simulink model "AMT103"  (R2024b)
settings: Solver=FixedStepAuto  StartTime=0.0  StopTime=inf  FixedStep=0.001  RelTol=1e-3  EnableMultiTasking=on
libraries: stm32f4xxblockslib x3, stm32g4xxblockslib x3, simulink x1
settings Model: STM32="{\"DigitalPortRead\":[{\"ID\":\"e:8\"},{\"ID\":\"e:9\"},{\"ID\":\"e:38\"},{\"ID\":\"e:39\"},{\"ID\":\"AMT103:38\"},{\"ID\":\"AMT103:9\"},{\"ID\":\"AMT103:8\"}],\"EncoderBlockForG4\":[{\"ID\":\"e:26\"},{\"ID\":\"e:27\"},{\"ID\":\"e:28\"},{\"ID\":\"AMT103:26\"},{\"ID\":\"AMT103:27\"},{\"ID\":\"AMT103:28\"}]}"  SimulationMode=external  Creator=gamen  LastModifiedBy=gamen
settings OptimizationCC: DefaultParameterBehavior=Inlined  EnhancedBackFolding=on  PassReuseOutputArgsAs=Individual arguments  ZeroExternalMemoryAtStartup=off  ZeroInternalMemoryAtStartup=off  MaxStackSize=512  OptimizeBlockOrder=speed  DifferentSizesBufferReuse=on  OptimizationCustomize=off  EfficientTunableParamExpr=on
settings DebuggingCC: ParameterTunabilityLossMsg=error
settings HardwareCC: ProdBitPerPointer=32  ProdBitPerSizeT=32  ProdBitPerPtrDiffT=32  ProdLargestAtomicInteger=Long  ProdLargestAtomicFloat=Double  ProdWordSize=32  ProdLongLongMode=on  ProdHWDeviceType=ARM Compatible->ARM Cortex-M
settings SFSimCC: MATLABDynamicMemAlloc=off
settings RTWCC: Description=Embedded Coder  SystemTargetFile=ert.tlc  HardwareBoard=STM32G4xx Based  TemplateMakefile=ert_default_tmf  Toolchain=GNU Tools for ARM Embedded Processors
settings CodeAppCC: ForceParamTrailComments=on  IgnoreCustomStorageClasses=off  OperatorAnnotations=on  SimulinkDataObjDesc=on  SFDataObjDesc=on  InsertBlockDesc=on
settings ERTTargetCC: TargetLangStandard=C99 (ISO)  CodeReplacementLibrary=ARM Cortex-M  ExtModeTransport=3  ExtModeStaticAlloc=on  ExtModeStaticAllocSize=2048  ExtModeMexFile=ext_xcp  ExtModeIntrfLevel=Level2 - Open

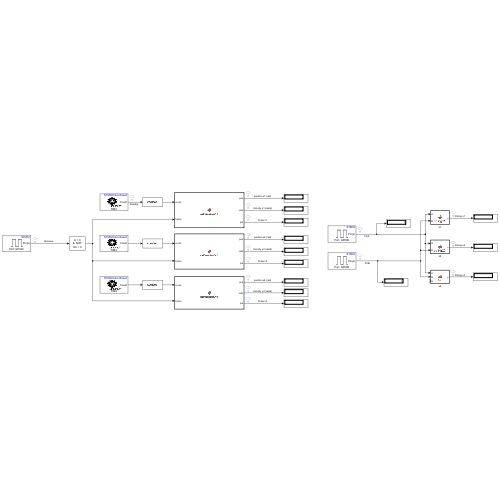
[thumbnail: Simulink's stored preview of the top-level diagram]
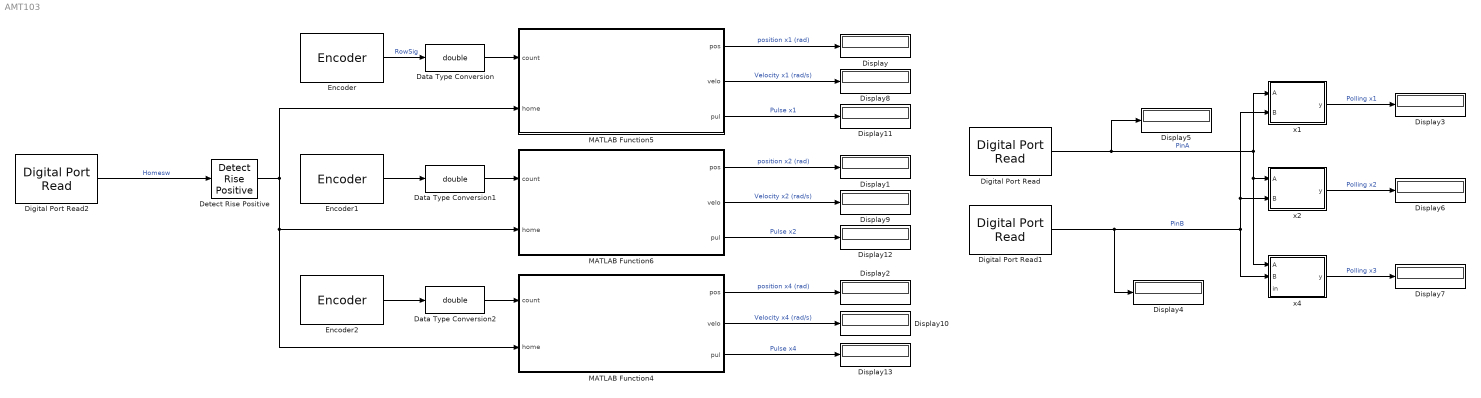
== system AMT103 ==
  Data Type Conversion : DataTypeConversion  OutDataTypeStr=double  SaturateOnIntegerOverflow=off  RndMeth=Floor
  Data Type Conversion1 : DataTypeConversion  OutDataTypeStr=double  SaturateOnIntegerOverflow=off  RndMeth=Floor
  Data Type Conversion2 : DataTypeConversion  OutDataTypeStr=double  SaturateOnIntegerOverflow=off  RndMeth=Floor
  Detect Rise Positive : simulink/Logic and Bit Operations/Detect Rise Positive  vinit=0  OutDataTypeStr=boolean
  Digital Port Read : stm32f4xxblockslib/Digital Port Read  PortName=GPIOB  PinNumber=[4]  ReadOperation=on  IOAsArray=on  SampleTime=-1  EnableSimPort=off  hoistedMaskSrc=ECSoC/ECSimCodegen/Digital Port Read
      settings: LibrarySourceBlock=stm32g4xxblockslib/Digital Port Read
  Digital Port Read1 : stm32f4xxblockslib/Digital Port Read  PortName=GPIOB  PinNumber=[5]  ReadOperation=on  IOAsArray=on  SampleTime=-1  EnableSimPort=off  hoistedMaskSrc=ECSoC/ECSimCodegen/Digital Port Read
      settings: LibrarySourceBlock=stm32g4xxblockslib/Digital Port Read
  Digital Port Read2 : stm32f4xxblockslib/Digital Port Read  PortName=GPIOC  PinNumber=[13]  ReadOperation=on  IOAsArray=on  SampleTime=-1  EnableSimPort=off  hoistedMaskSrc=ECSoC/ECSimCodegen/Digital Port Read
      settings: LibrarySourceBlock=stm32g4xxblockslib/Digital Port Read
  Display{,1..13} (14 alike) : Display
  Encoder : stm32g4xxblockslib/Encoder  TimerModule=TIM3  EnableResetInput=off  OutputCountAfterFirstIndex=off  OutputValidIndex=off  OutputDirection=off  OutputStatus=off  SampleTime=-1
  Encoder1 : stm32g4xxblockslib/Encoder  TimerModule=TIM4  EnableResetInput=off  OutputCountAfterFirstIndex=off  OutputValidIndex=off  OutputDirection=off  OutputStatus=off  SampleTime=-1
  Encoder2 : stm32g4xxblockslib/Encoder  TimerModule=TIM8  EnableResetInput=off  OutputCountAfterFirstIndex=off  OutputValidIndex=off  OutputDirection=off  OutputStatus=off  SampleTime=-1
  MATLAB Function4 : MATLAB Function  TreatAsAtomicUnit=on
  MATLAB Function5 : MATLAB Function  TreatAsAtomicUnit=on
  MATLAB Function6 : MATLAB Function  TreatAsAtomicUnit=on
  x1 : MATLAB Function  TreatAsAtomicUnit=on
  x2 : MATLAB Function  TreatAsAtomicUnit=on
  x4 : MATLAB Function  TreatAsAtomicUnit=on
  wires:
  MATLAB Function6/1(pos) -> Display1/1  "position x2 (rad)"
  Encoder2/1 -> Data Type Conversion2/1
  x2/1(y) -> Display6/1  "Polling x2"
  x4/1(y) -> Display7/1  "Polling x3"
  MATLAB Function5/1(pos) -> Display/1  "position x1 (rad)"
  MATLAB Function6/2(velo) -> Display9/1  "Velocity x2 (rad/s)"
  Data Type Conversion/1 -> MATLAB Function5/1(count)
  MATLAB Function4/3(pul) -> Display13/1  "Pulse x4"
  Encoder/1 -> Data Type Conversion/1  "RowSig"
  Data Type Conversion2/1 -> MATLAB Function4/1(count)
  Digital Port Read1/1 -> x1/2(B), x2/2(B), x4/2(B), Display4/1  "PinB"
  Data Type Conversion1/1 -> MATLAB Function6/1(count)
  MATLAB Function4/1(pos) -> Display2/1  "position x4 (rad)"
  MATLAB Function6/3(pul) -> Display12/1  "Pulse x2"
  Digital Port Read/1 -> Display5/1, x1/1(A), x4/1(A), x2/1(A)  "PinA"
  x1/1(y) -> Display3/1  "Polling x1"
  MATLAB Function5/2(velo) -> Display8/1  "Velocity x1 (rad/s)"
  MATLAB Function4/2(velo) -> Display10/1  "Velocity x4 (rad/s)"
  MATLAB Function5/3(pul) -> Display11/1  "Pulse x1"
  Encoder1/1 -> Data Type Conversion1/1
  Digital Port Read2/1 -> Detect Rise Positive/1  "Homesw"
  Detect Rise Positive/1 -> MATLAB Function5/2(home), MATLAB Function4/2(home), MATLAB Function6/2(home)

== matlab function AMT103/x1 ==
  data: A input; y output; B input
function y =  pollingX1(A, B)
    persistent c stageA
    if isempty(c)
        c = 0;
        stageA = 1;
    end

    if A == 0 && stageA
        stageA = 0;
        c = c + 2 * B - 1;
    elseif A == 1
        stageA = 1;
    end

    y = c;
end

== matlab function AMT103/x2 ==
  data: A input; y output; B input
function y = pollingX2(A, B)
    persistent c stageA
    if isempty(c)
        c = 0;
        stageA = 1;
    end

    if A == 0 && stageA
        stageA = 0;
        c = c + 2 * B - 1;
    elseif A == 1 && ~stageA
        stageA = 1;
        c = c + 1 - 2 * B;
    end

    y = c;
end

== matlab function AMT103/x4 ==
  data: A input; y output; B input; in input
function y = fcn(A,B,in)
persistent c
persistent stageA
persistent stageB
if isempty(c)
   c = 0;
   stageA=1;
   stageB=1;
end
if in==1
    c=0;
end
if A==0 && stageA==1
    stageA=0;
    if B==1
        c=c+1;
    else
        c=c-1;
    end
else
    if A==1 && stageA==0
        stageA=1;
        if B==0
            c=c+1;
        else
            c=c-1;
        end
    end
end

if B==0 && stageB==1
    stageB=0;
    if A==0
        c=c+1;
    else
        c=c-1;
    end
else
    if B==1 && stageB==0
        stageB=1;
        if A==1
            c=c+1;
        else
            c=c-1;
        end
    end
end


y = c;

== matlab function AMT103/MATLAB Function4 ==
  data: count input; pos output; velo output; pul output; home input
function [pos, velo, pul] = calFunctionX4(count, home)
    persistent pulse lastpulse lastrad home_position;
    
    if isempty(pulse)
        pulse = 0;
        lastpulse = 0;
        lastrad = 0;
        home_position = 0;
    end
    
    pulse_diff = count - lastpulse;
    if abs(pulse_diff) > 10000
        pulse = pulse + (8258.68 * sign(pulse_diff) - pulse_diff);
    else
        pulse = pulse + pulse_diff;
    end
    
    if home == 1
        home_position = pulse;
    end

    pul = pulse - home_position;
    pos = pul * (2 * pi / 96);
    velo = (pos - lastrad) / 0.1;
    
    lastpulse = count;
    lastrad = pos;
end

== matlab function AMT103/MATLAB Function5 ==
  data: count input; pos output; velo output; pul output; home input
function [pos, velo, pul] = calFunctionX1(count, home)
    persistent pulse lastpulse lastrad home_position;
    
    if isempty(pulse)
        pulse = 0;
        lastpulse = 0;
        lastrad = 0;
        home_position = 0;
    end
    
    pulse_diff = count - lastpulse;
    if abs(pulse_diff) > 10000
        pulse = pulse + (2064.67 * sign(pulse_diff) - pulse_diff);
    else
        pulse = pulse + pulse_diff;
    end
    
    if home == 1
        home_position = pulse;
    end

    pul = pulse - home_position;
    pos = pul * (2 * pi / 24);
    velo = (pos - lastrad) / 0.1;
    
    lastpulse = count;
    lastrad = pos;
end

== matlab function AMT103/MATLAB Function6 ==
  data: count input; pos output; velo output; pul output; home input
function [pos, velo, pul] = calFunctionX2(count, home)
    persistent pulse lastpulse lastrad home_position;
    
    if isempty(pulse)
        pulse = 0;
        lastpulse = 0;
        lastrad = 0;
        home_position = 0;
    end
    
    pulse_diff = count - lastpulse;
    if abs(pulse_diff) > 10000
        pulse = pulse + (4129.34 * sign(pulse_diff) - pulse_diff);
    else
        pulse = pulse + pulse_diff;
    end
    
    if home == 1
        home_position = pulse;
    end

    pul = pulse - home_position;
    pos = pul * (2 * pi / 48);
    velo = (pos - lastrad) / 0.1;
    
    lastpulse = count;
    lastrad = pos;
end
